simulink model "TractiveSystemTemperatures"  (R2024b)
settings: Solver=FixedStepAuto  StartTime=0.0  StopTime=10.0  RelTol=1e-3  EnableMultiTasking=on
settings Model: DataDictionary=Master_Dictionary.sldd  EnableAccessToBaseWorkspace=off  Creator=torni  LastModifiedBy=Will
settings OptimizationCC: DefaultParameterBehavior=Inlined  EnhancedBackFolding=on  PassReuseOutputArgsAs=Individual arguments  ZeroExternalMemoryAtStartup=off  ZeroInternalMemoryAtStartup=off  MaxStackSize=8192  OptimizeBlockOrder=speed  DifferentSizesBufferReuse=on  OptimizationCustomize=off  EfficientTunableParamExpr=on
settings DebuggingCC: ParameterTunabilityLossMsg=error
settings HardwareCC: ProdBitPerPointer=32  ProdBitPerSizeT=32  ProdBitPerPtrDiffT=32  ProdLargestAtomicInteger=Long  ProdLargestAtomicFloat=Double  ProdWordSize=32  ProdLongLongMode=on  ProdHWDeviceType=ARM Compatible->ARM Cortex-M
settings SFSimCC: MATLABDynamicMemAlloc=off
settings RTWCC: Description=Embedded Coder  SystemTargetFile=ert.tlc  HardwareBoard=STM32H7xx Based (Single-core)  TemplateMakefile=ert_default_tmf  Toolchain=GNU Tools for ARM Embedded Processors
settings CodeAppCC: ForceParamTrailComments=on  IgnoreCustomStorageClasses=off  OperatorAnnotations=on  SimulinkDataObjDesc=on  SFDataObjDesc=on  InsertBlockDesc=on
settings ERTTargetCC: TargetLangStandard=C99 (ISO)  CodeReplacementLibrary=ARM Cortex-M  ExtModeTransport=3  ExtModeStaticAlloc=on  ExtModeStaticAllocSize=2048  ExtModeMexFile=ext_xcp  ExtModeIntrfLevel=Level2 - Open

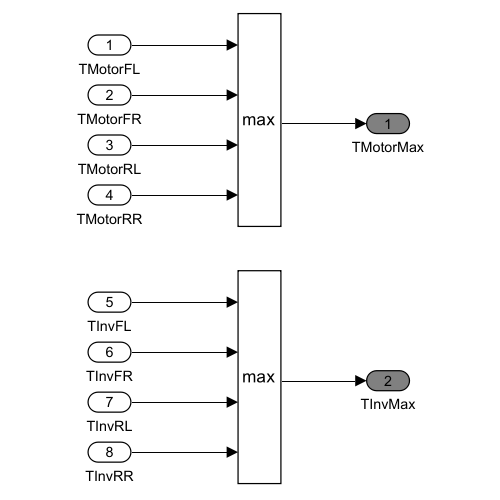
[thumbnail: Simulink's stored preview of the top-level diagram]
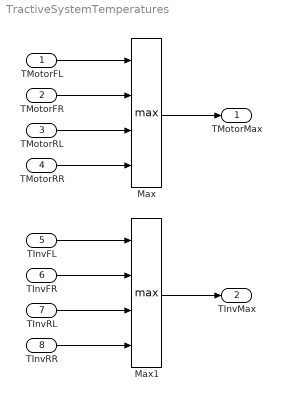
== system TractiveSystemTemperatures ==
  TMotorFL : Inport  OutDataTypeStr=double
  "TMotorFR " : Inport  Port=2  OutDataTypeStr=double
  TMotorRL : Inport  Port=3  OutDataTypeStr=double
  TMotorRR : Inport  Port=4  OutDataTypeStr=double
  TInvFL : Inport  Port=5  OutDataTypeStr=double
  TInvFR : Inport  Port=6  OutDataTypeStr=double
  TInvRL : Inport  Port=7  OutDataTypeStr=double
  TInvRR : Inport  Port=8  OutDataTypeStr=double
  Max : MinMax  Function=max  Inputs=4
  Max1 : MinMax  Function=max  Inputs=4
  TMotorMax : Outport  OutDataTypeStr=double  VectorParamsAs1DForOutWhenUnconnected=off
  TInvMax : Outport  Port=2  OutDataTypeStr=double  VectorParamsAs1DForOutWhenUnconnected=off
  wires:
  TMotorFL/1 -> Max/1
  TMotorRR/1 -> Max/4
  TMotorRL/1 -> Max/3
  "TMotorFR "/1 -> Max/2
  Max/1 -> TMotorMax/1
  Max1/1 -> TInvMax/1
  TInvFR/1 -> Max1/2
  TInvRL/1 -> Max1/3
  TInvRR/1 -> Max1/4
  TInvFL/1 -> Max1/1
